simulink model "AirSys_AirTemp"  (R2016b)
settings: configuration reference "CodeGenConfigSet" (kept outside this file)
settings Model: Creator=lenovo  LastModifiedBy=Administrator
settings ConfigSetRef: SourceLocation=Base Workspace

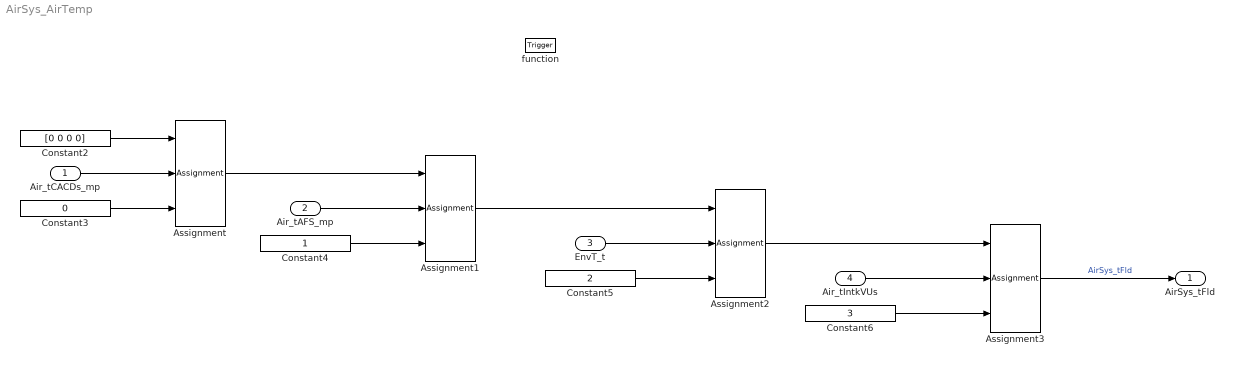
== system AirSys_AirTemp ==
  Air_tCACDs_mp : Inport  Tag=deg  Description=Charge-air temperature downstream from charge-air cooler  OutMin=-200  OutMax=200  OutDataTypeStr=Temp_deg
  Air_tAFS_mp : Inport  Tag=deg  Description=Induction air temperature at the HFM  Port=2  OutMin=-200  OutMax=200  OutDataTypeStr=Temp_deg
  EnvT_t : Inport  Tag=deg  Description=Environmental temperature  Port=3  OutMin=-200  OutMax=200  OutDataTypeStr=Temp_deg
  Air_tIntkVUs : Inport  Tag=deg  Description=Intake air temperature upstream of the inlet valve  Port=4  OutMin=-200  OutMax=200  OutDataTypeStr=Temp_deg
  function : TriggerPort  TriggerType=function-call  VariantControl=Variant
  Assignment : Assignment  IndexMode=Zero-based  DiagnosticForDimensions=Warning  IndexOptions=Index vector (port)  Indices=1  OutputSizes=1
  Assignment1 : Assignment  IndexMode=Zero-based  DiagnosticForDimensions=Warning  IndexOptions=Index vector (port)  Indices=1  OutputSizes=1
  Assignment2 : Assignment  IndexMode=Zero-based  DiagnosticForDimensions=Warning  IndexOptions=Index vector (port)  Indices=4  OutputSizes=1
  Assignment3 : Assignment  IndexMode=Zero-based  DiagnosticForDimensions=Warning  IndexOptions=Index vector (port)  Indices=4  OutputSizes=1
  Constant2 : Constant  Value=[0 0 0 0]  OutDataTypeStr=Inherit: Inherit via back propagation
  Constant3 : Constant  Value=0  OutDataTypeStr=uint8
  Constant4 : Constant  OutDataTypeStr=uint8
  Constant5 : Constant  Value=2  OutDataTypeStr=uint8
  Constant6 : Constant  Value=3  OutDataTypeStr=uint8
  AirSys_tFld : Outport  Tag=deg  Description=Engine temperature field  OutMin=-1000  OutMax=1000  OutDataTypeStr=Temp_deg
  wires:
  Constant6/1 -> Assignment3/3
  Assignment2/1 -> Assignment3/1
  Constant5/1 -> Assignment2/3
  Assignment1/1 -> Assignment2/1
  Constant4/1 -> Assignment1/3
  Assignment/1 -> Assignment1/1
  Constant3/1 -> Assignment/3
  Constant2/1 -> Assignment/1
  Air_tCACDs_mp/1 -> Assignment/2
  Assignment3/1 -> AirSys_tFld/1  "AirSys_tFld"
  EnvT_t/1 -> Assignment2/2
  Air_tIntkVUs/1 -> Assignment3/2
  Air_tAFS_mp/1 -> Assignment1/2
